simulink model "algeb1"  (Simulink 2.00)
settings: Solver=ode45  StartTime=0.0  StopTime=10.0  MaxStep=0.1  RelTol=1e-3  AbsTol=1e-6
settings Model: Refine=3  InitialStep=0.01  ConsistencyChecking=off

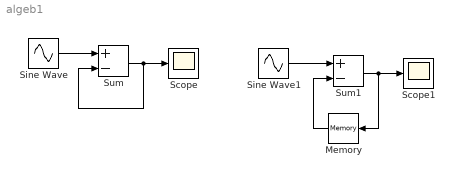
== system algeb1 ==
  Memory : Memory  Orientation=left  X0=0  InheritSampleTime=off
  Scope : Scope
      settings: TickLabels=on  TimeRange=auto  YMin=-5  YMax=5  SaveToWorkspace=off  SaveName=ScopeData
  Scope1 : Scope
      settings: TickLabels=on  TimeRange=auto  YMin=-5  YMax=5  SaveToWorkspace=off  SaveName=ScopeData
  Sine Wave : Sin  Amplitude=1  Frequency=1  Phase=0  SampleTime=-1
  Sine Wave1 : Sin  Amplitude=1  Frequency=1  Phase=0  SampleTime=-1
  Sum : Sum  Inputs=+-
  Sum1 : Sum  Inputs=+-
  wires:
  Sine Wave/1 -> Sum/1
  Sum/1 -> Scope/1, Sum/2
  Sine Wave1/1 -> Sum1/1
  Memory/1 -> Sum1/2
  Sum1/1 -> Scope1/1, Memory/1
